simulink model "bpsk_receiver"  (R2020a)
settings: Solver=VariableStepAuto  StartTime=0.0  StopTime=10000/3.2e6  RelTol=1e-3
InitFcn:
  | setup_bpsk_receiver
undefined symbols (not defined in the file): AXI4, designMultirateFIR, fir_bbuf, Lite, tx_data, xlfda_numerator
libraries: xbsIndex_r4 x367, hdlsllib x15, dspmlti4 x8, xrbsSSR_Library x6, dspswit3 x4, dspsigops x2, commrandsrc3 x1, simulink x1
(part 1 of 4)
settings Model: SimulationMode=accelerator  Creator=david  LastModifiedBy=david
settings SFSimCC: CustomCodeUndefinedFunction=UseInterfaceOnly

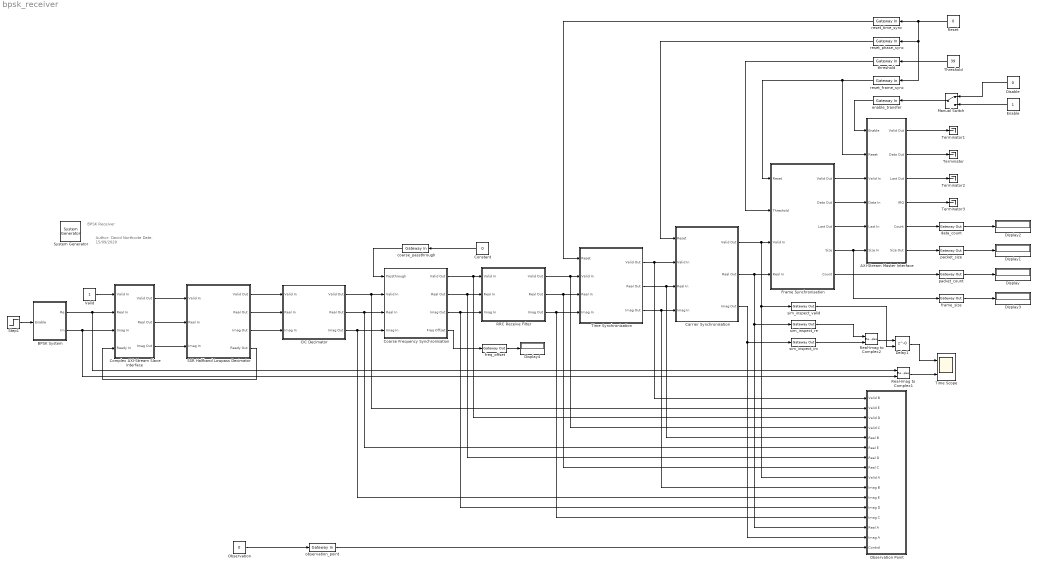
== system bpsk_receiver ==
  note: Author: 	David Northcote
      | Date: 	15/09/2020
  note: BPSK Receiver
  " System Generator" : xbsIndex_r4/ System Generator  Tag=genX  xilinxfamily=zynquplusRFSOC  part=xczu28dr  speed=-2-e  package=ffvg1517  synthesis_tool=Vivado  clock_wrapper=Clock Enables  directory=./netlist  proj_type=Vivado  Synth_file=Vivado Synthesis Defaults  Impl_file=Vivado Implementation Defaults  testbench=off  simulink_period=1/64e6  sysclk_period=(1/64e6)*1e9  dcm_input_clock_period=10  incr_netlist=off  trim_vbits=Everywhere in SubSystem  dbl_ovrd=According to Block Masks  core_generation=According to Block Masks  run_coregen=off  deprecated_control=off  eval_field=0  block_type=sysgen
  AXI-Stream Master Interface : Subsystem
  BPSK System : Subsystem
  CIC Decimator : Subsystem
  Carrier Synchronisation : Subsystem
  Coarse Frequency Synchronisation : Subsystem
  Complex AXI-Stream Slave Interface : Subsystem
  Constant : Constant  Value=0  SampleTime=-1
  Delay1 : Delay  DelayLength=0  ShowEnablePort=on
      settings: InputPortMap=u0,e6
  Disable : Constant  Value=0  OutDataTypeStr=boolean  SampleTime=-1
  Display{,1..4} (5 alike) : Display
  Enable : Constant  OutDataTypeStr=boolean  SampleTime=-1
  Frame Synchronisation : Subsystem
  Manual Switch : ManualSwitch
  Observation : Constant  Value=0  OutDataTypeStr=uint32  SampleTime=-1
  Observation Point : Subsystem
  RRC Receive Filter : Subsystem
  Real-Imag to Complex1 : RealImagToComplex
  Real-Imag to Complex2 : RealImagToComplex
  Reset : Constant  Value=0  OutDataTypeStr=boolean  SampleTime=-1
  SSR Halfband Lowpass Decimator : Subsystem
  Step1 : Step  Time=2/12.5e3  SampleTime=1/12.5e3
  Terminator{,1..3} (4 alike) : Terminator
  Threshold : Constant  Value=39  OutDataTypeStr=uint32  SampleTime=-1
  Time Scope : Scope  NumInputPorts=2
  Time Synchronisation : Subsystem
  Valid : Constant  OutDataTypeStr=boolean  SampleTime=1/64e6
  coarse_passthrough : xbsIndex_r4/Gateway In  gui_display_data_type=Boolean  arith_type=Boolean  n_bits=16  bin_pt=14  preci_type=Single  exp_width=8  frac_width=24  rows=1  columns=1  quantization="Round  (unbiased: +/- Inf)"  overflow=Saturate  period=1/12.8e6  UseAsADC=off  ADCChannel='1'  interface=AXI4-Lite  automatic_assignment=off  address_offset=44  intf_name=''  intf_description=''  default_value=0  timing_constraint=None  locs_specified=off  LOCs={}  io_standard={}  inherit_from_input=off  hdl_port=on  dbl_ovrd=off  block_type=gatewayin
  data_count : xbsIndex_r4/Gateway Out  inherit_from_input=on  hdl_port=on  rows=1  columns=1  UseAsDAC=off  DACChannel='1'  interface=AXI4-Lite  automatic_assignment=off  address_offset=32  intf_name=''  intf_description=''  timing_constraint=None  locs_specified=off  LOCs={}  io_standard={}  block_type=gatewayout
  enable_transfer : xbsIndex_r4/Gateway In  gui_display_data_type=Boolean  arith_type=Boolean  n_bits=16  bin_pt=14  preci_type=Single  exp_width=8  frac_width=24  rows=1  columns=1  quantization="Round  (unbiased: +/- Inf)"  overflow=Saturate  period=1/64e6  UseAsADC=off  ADCChannel='1'  interface=AXI4-Lite  automatic_assignment=off  address_offset=28  intf_name=''  intf_description=''  default_value=0  timing_constraint=None  locs_specified=off  LOCs={}  io_standard={}  inherit_from_input=off  hdl_port=on  dbl_ovrd=off  block_type=gatewayin
  frame_size : xbsIndex_r4/Gateway Out  inherit_from_input=on  hdl_port=on  rows=1  columns=1  UseAsDAC=off  DACChannel='1'  interface=AXI4-Lite  automatic_assignment=off  address_offset=16  intf_name=''  intf_description=''  timing_constraint=None  locs_specified=off  LOCs={}  io_standard={}  block_type=gatewayout
  freq_offset : xbsIndex_r4/Gateway Out  inherit_from_input=on  hdl_port=on  rows=1  columns=1  UseAsDAC=off  DACChannel='1'  interface=AXI4-Lite  automatic_assignment=off  address_offset=40  intf_name=''  intf_description=''  timing_constraint=None  locs_specified=off  LOCs={}  io_standard={}  block_type=gatewayout
  observation_point : xbsIndex_r4/Gateway In  gui_display_data_type=Fixed-point  arith_type=Unsigned  n_bits=32  bin_pt=0  preci_type=Single  exp_width=8  frac_width=24  rows=1  columns=1  quantization="Round  (unbiased: +/- Inf)"  overflow=Saturate  period=1/64e6  UseAsADC=off  ADCChannel='1'  interface=AXI4-Lite  automatic_assignment=off  address_offset=36  intf_name=''  intf_description=''  default_value=0  timing_constraint=None  locs_specified=off  LOCs={}  io_standard={}  inherit_from_input=off  hdl_port=on  dbl_ovrd=off  block_type=gatewayin
  packet_count : xbsIndex_r4/Gateway Out  inherit_from_input=on  hdl_port=on  rows=1  columns=1  UseAsDAC=off  DACChannel='1'  interface=AXI4-Lite  automatic_assignment=off  address_offset=24  intf_name=''  intf_description=''  timing_constraint=None  locs_specified=off  LOCs={}  io_standard={}  block_type=gatewayout
  packet_size : xbsIndex_r4/Gateway Out  inherit_from_input=on  hdl_port=on  rows=1  columns=1  UseAsDAC=off  DACChannel='1'  interface=AXI4-Lite  automatic_assignment=off  address_offset=20  intf_name=''  intf_description=''  timing_constraint=None  locs_specified=off  LOCs={}  io_standard={}  block_type=gatewayout
  reset_frame_sync : xbsIndex_r4/Gateway In  gui_display_data_type=Boolean  arith_type=Boolean  n_bits=16  bin_pt=14  preci_type=Single  exp_width=8  frac_width=24  rows=1  columns=1  quantization="Round  (unbiased: +/- Inf)"  overflow=Saturate  period=1/3.2e6  UseAsADC=off  ADCChannel='1'  interface=AXI4-Lite  automatic_assignment=off  address_offset=8  intf_name=''  intf_description=''  default_value=1  timing_constraint=None  locs_specified=off  LOCs={}  io_standard={}  inherit_from_input=off  hdl_port=on  dbl_ovrd=off  block_type=gatewayin
  reset_phase_sync : xbsIndex_r4/Gateway In  gui_display_data_type=Boolean  arith_type=Boolean  n_bits=16  bin_pt=14  preci_type=Single  exp_width=8  frac_width=24  rows=1  columns=1  quantization="Round  (unbiased: +/- Inf)"  overflow=Saturate  period=1/3.2e6  UseAsADC=off  ADCChannel='1'  interface=AXI4-Lite  automatic_assignment=off  address_offset=4  intf_name=''  intf_description=''  default_value=1  timing_constraint=None  locs_specified=off  LOCs={}  io_standard={}  inherit_from_input=off  hdl_port=on  dbl_ovrd=off  block_type=gatewayin
  reset_time_sync : xbsIndex_r4/Gateway In  gui_display_data_type=Boolean  arith_type=Boolean  n_bits=16  bin_pt=14  preci_type=Single  exp_width=8  frac_width=24  rows=1  columns=1  quantization="Round  (unbiased: +/- Inf)"  overflow=Saturate  period=1/3.2e6  UseAsADC=off  ADCChannel='1'  interface=AXI4-Lite  automatic_assignment=off  address_offset=0  intf_name=''  intf_description=''  default_value=1  timing_constraint=None  locs_specified=off  LOCs={}  io_standard={}  inherit_from_input=off  hdl_port=on  dbl_ovrd=off  block_type=gatewayin
  sim_inspect_im : xbsIndex_r4/Gateway Out  inherit_from_input=on  hdl_port=off  rows=1  columns=1  UseAsDAC=off  DACChannel='1'  interface=None  automatic_assignment=on  address_offset=hex2dec('00')  intf_name=''  intf_description=''  timing_constraint=None  locs_specified=off  LOCs={}  io_standard={}  block_type=gatewayout
  sim_inspect_re : xbsIndex_r4/Gateway Out  inherit_from_input=on  hdl_port=off  rows=1  columns=1  UseAsDAC=off  DACChannel='1'  interface=None  automatic_assignment=on  address_offset=hex2dec('00')  intf_name=''  intf_description=''  timing_constraint=None  locs_specified=off  LOCs={}  io_standard={}  block_type=gatewayout
  sim_inspect_valid : xbsIndex_r4/Gateway Out  inherit_from_input=on  hdl_port=off  rows=1  columns=1  UseAsDAC=off  DACChannel='1'  interface=None  automatic_assignment=on  address_offset=hex2dec('00')  intf_name=''  intf_description=''  timing_constraint=None  locs_specified=off  LOCs={}  io_standard={}  block_type=gatewayout
  threshold : xbsIndex_r4/Gateway In  gui_display_data_type=Fixed-point  arith_type=Unsigned  n_bits=32  bin_pt=0  preci_type=Single  exp_width=8  frac_width=24  rows=1  columns=1  quantization="Round  (unbiased: +/- Inf)"  overflow=Saturate  period=1/3.2e6  UseAsADC=off  ADCChannel='1'  interface=AXI4-Lite  automatic_assignment=off  address_offset=12  intf_name=''  intf_description=''  default_value=39  timing_constraint=None  locs_specified=off  LOCs={}  io_standard={}  inherit_from_input=off  hdl_port=on  dbl_ovrd=off  block_type=gatewayin
  wires:
  reset_time_sync/1 -> Time Synchronisation/1(Reset)
  Reset/1 -> reset_phase_sync/1, reset_frame_sync/1, reset_time_sync/1
  Time Synchronisation/1(Valid Out) -> Observation Point/1(Valid B), Carrier Synchronisation/2(Valid In)
  Time Synchronisation/2(Real Out) -> Carrier Synchronisation/3(Real In), Observation Point/5(Real B)
  Time Synchronisation/3(Imag Out) -> Carrier Synchronisation/4(Imag In), Observation Point/10(Imag B)
  reset_phase_sync/1 -> Carrier Synchronisation/1(Reset)
  Carrier Synchronisation/2(Real Out) -> sim_inspect_re/1, Observation Point/14(Real A), Frame Synchronisation/4(Real In)
  Carrier Synchronisation/1(Valid Out) -> sim_inspect_valid/1, Observation Point/9(Valid A), Frame Synchronisation/3(Valid In)
  threshold/1 -> Frame Synchronisation/2(Threshold)
  reset_frame_sync/1 -> AXI-Stream Master Interface/2(Reset), Frame Synchronisation/1(Reset)
  Threshold/1 -> threshold/1
  Carrier Synchronisation/3(Imag Out) -> sim_inspect_im/1, Observation Point/15(Imag A)
  Frame Synchronisation/5(Count) -> packet_count/1
  Real-Imag to Complex1/1 -> Time Scope/2
  sim_inspect_valid/1 -> Delay1/2
  Real-Imag to Complex2/1 -> Delay1/1
  sim_inspect_re/1 -> Real-Imag to Complex2/1
  sim_inspect_im/1 -> Real-Imag to Complex2/2
  Delay1/1 -> Time Scope/1
  Frame Synchronisation/3(Last Out) -> AXI-Stream Master Interface/5(Last In)
  packet_count/1 -> Display/1
  packet_size/1 -> Display1/1
  AXI-Stream Master Interface/6(Size Out) -> packet_size/1
  Frame Synchronisation/4(Size) -> frame_size/1, AXI-Stream Master Interface/6(Size In)
  enable_transfer/1 -> AXI-Stream Master Interface/1(Enable)
  AXI-Stream Master Interface/5(Count) -> data_count/1
  data_count/1 -> Display2/1
  AXI-Stream Master Interface/2(Data Out) -> Terminator/1
  AXI-Stream Master Interface/1(Valid Out) -> Terminator1/1
  AXI-Stream Master Interface/3(Last Out) -> Terminator2/1
  AXI-Stream Master Interface/4(IRQ) -> Terminator3/1
  Frame Synchronisation/1(Valid Out) -> AXI-Stream Master Interface/3(Valid In)
  Frame Synchronisation/2(Data Out) -> AXI-Stream Master Interface/4(Data In)
  Manual Switch/1 -> enable_transfer/1
  Disable/1 -> Manual Switch/1
  Enable/1 -> Manual Switch/2
  Complex AXI-Stream Slave Interface/3(Imag Out) -> SSR Halfband Lowpass Decimator/3(Imag In)
  Complex AXI-Stream Slave Interface/2(Real Out) -> SSR Halfband Lowpass Decimator/2(Real In)
  Complex AXI-Stream Slave Interface/1(Valid Out) -> SSR Halfband Lowpass Decimator/1(Valid In)
  SSR Halfband Lowpass Decimator/4(Ready Out) -> Complex AXI-Stream Slave Interface/4(Ready In)
  Valid/1 -> Complex AXI-Stream Slave Interface/1(Valid In)
  Step1/1 -> BPSK System/1(Enable)
  BPSK System/2(Im) -> Complex AXI-Stream Slave Interface/3(Imag In), Real-Imag to Complex1/2
  BPSK System/1(Re) -> Complex AXI-Stream Slave Interface/2(Real In), Real-Imag to Complex1/1
  RRC Receive Filter/1(Valid Out) -> Time Synchronisation/2(Valid In), Observation Point/4(Valid C)
  RRC Receive Filter/2(Real Out) -> Time Synchronisation/3(Real In), Observation Point/8(Real C)
  RRC Receive Filter/3(Imag Out) -> Time Synchronisation/4(Imag In), Observation Point/13(Imag C)
  SSR Halfband Lowpass Decimator/2(Real Out) -> CIC Decimator/2(Real In)
  SSR Halfband Lowpass Decimator/3(Imag Out) -> CIC Decimator/3(Imag In)
  Observation/1 -> observation_point/1
  observation_point/1 -> Observation Point/16(Control)
  frame_size/1 -> Display3/1
  CIC Decimator/1(Valid Out) -> Coarse Frequency Synchronisation/2(Valid In), Observation Point/2(Valid E)
  CIC Decimator/2(Real Out) -> Coarse Frequency Synchronisation/3(Real In), Observation Point/6(Real E)
  CIC Decimator/3(Imag Out) -> Coarse Frequency Synchronisation/4(Imag In), Observation Point/11(Imag E)
  Coarse Frequency Synchronisation/1(Valid Out) -> Observation Point/3(Valid D), RRC Receive Filter/1(Valid In)
  Coarse Frequency Synchronisation/2(Real Out) -> Observation Point/7(Real D), RRC Receive Filter/2(Real In)
  Coarse Frequency Synchronisation/3(Imag Out) -> Observation Point/12(Imag D), RRC Receive Filter/3(Imag In)
  freq_offset/1 -> Display4/1
  Coarse Frequency Synchronisation/4(Freq Offset) -> freq_offset/1
  Constant/1 -> coarse_passthrough/1
  coarse_passthrough/1 -> Coarse Frequency Synchronisation/1(Passthrough)
  SSR Halfband Lowpass Decimator/1(Valid Out) -> CIC Decimator/1(Valid In)

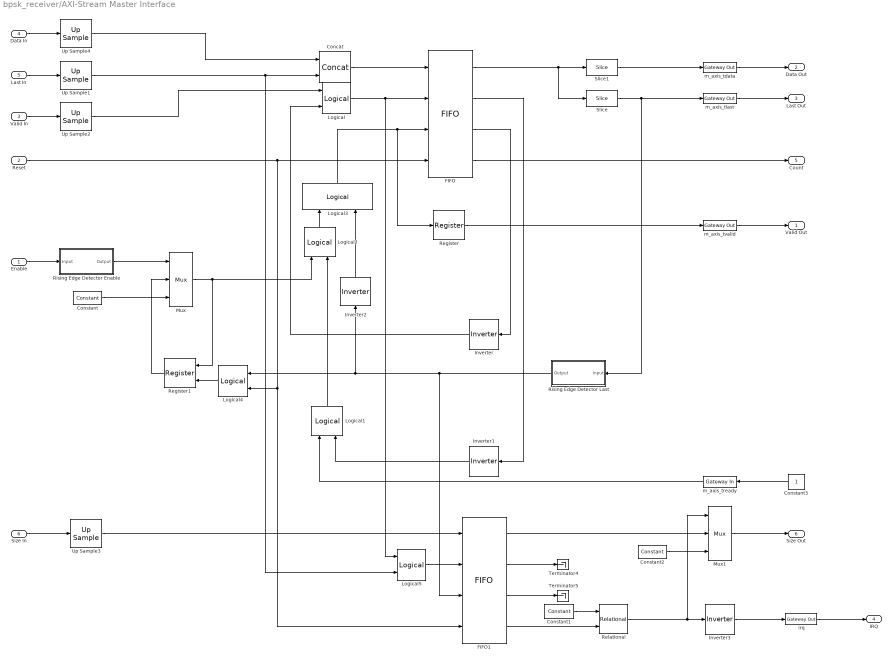
== system bpsk_receiver/AXI-Stream Master Interface ==
  Enable : Inport
  Reset : Inport  Port=2
  Valid In : Inport  Port=3
  Data In : Inport  Port=4
  Last In : Inport  Port=5
  Size In : Inport  Port=6
  Concat : xbsIndex_r4/Concat  num_inputs=2  dbl_ovrd=off  block_type=concat
  Constant : xbsIndex_r4/Constant  const=1.0  gui_display_data_type=Boolean  arith_type=Boolean  n_bits=16  bin_pt=14  preci_type=Single  exp_width=8  frac_width=24  explicit_period=off  period=1  equ=P=C  opselect=C  inp2=PCIN>>17  opr=+  inp1=P  carry=CIN  dbl_ovrd=off  block_type=constant
  Constant1 : xbsIndex_r4/Constant  const=0  gui_display_data_type=Fixed-point  arith_type=Unsigned  n_bits=1  bin_pt=0  preci_type=Single  exp_width=8  frac_width=24  explicit_period=off  period=1  equ=P=C  opselect=C  inp2=PCIN>>17  opr=+  inp1=P  carry=CIN  dbl_ovrd=off  block_type=constant
  Constant2 : xbsIndex_r4/Constant  const=0  gui_display_data_type=Fixed-point  arith_type=Unsigned  n_bits=8  bin_pt=0  preci_type=Single  exp_width=8  frac_width=24  explicit_period=off  period=1  equ=P=C  opselect=C  inp2=PCIN>>17  opr=+  inp1=P  carry=CIN  dbl_ovrd=off  block_type=constant
  Constant3 : Constant  SampleTime=1/64e6
  FIFO : xbsIndex_r4/FIFO  mem_type=Block RAM  performance_options=Standard_FIFO  embedded_registers=off  depth=4K  percent_nbits=1  rst=on  rst_latency=2  en=off  use_dcount=on  use_percent_full_port=off  use_almost_empty=off  almost_empty_thresh=2  use_almost_full=off  use_rd_rst_busy=off  use_wr_rst_busy=off  almost_full_thresh=14  explicit_period=off  dbl_ovrd=off  simulation_type=fast_sim  block_type=fifo
  FIFO1 : xbsIndex_r4/FIFO  mem_type=Block RAM  performance_options=First_Word_Fall_Through  embedded_registers=off  depth=4K  percent_nbits=1  rst=on  rst_latency=2  en=off  use_dcount=on  use_percent_full_port=off  use_almost_empty=off  almost_empty_thresh=2  use_almost_full=off  use_rd_rst_busy=off  use_wr_rst_busy=off  almost_full_thresh=14  explicit_period=off  dbl_ovrd=off  simulation_type=fast_sim  block_type=fifo
  Inverter{,1..3} (4 alike) : xbsIndex_r4/Inverter  en=off  latency=0  dbl_ovrd=off  block_type=inv
  Logical{,1..3,5} (5 alike) : xbsIndex_r4/Logical  logical_function=AND  inputs=2  en=off  latency=0  precision=Full  arith_type=Unsigned  n_bits=16  bin_pt=0  align_bp=on  dbl_ovrd=off  block_type=logical
  Logical4 : xbsIndex_r4/Logical  logical_function=OR  inputs=2  en=off  latency=0  precision=Full  arith_type=Unsigned  n_bits=16  bin_pt=0  align_bp=on  dbl_ovrd=off  block_type=logical
  Mux : xbsIndex_r4/Mux  inputs=2  en=off  latency=0  precision=Full  arith_type=Unsigned  n_bits=16  bin_pt=14  quantization=Truncate  overflow=Wrap  dbl_ovrd=off  block_type=mux
  Mux1 : xbsIndex_r4/Mux  inputs=2  en=off  latency=0  precision=Full  arith_type=Unsigned  n_bits=16  bin_pt=14  quantization=Truncate  overflow=Wrap  dbl_ovrd=off  block_type=mux
  Register : xbsIndex_r4/Register  init=0  rst=off  en=off  dbl_ovrd=off  block_type=register
  Register1 : xbsIndex_r4/Register  init=0  rst=on  en=off  dbl_ovrd=off  block_type=register
  Relational : xbsIndex_r4/Relational  mode=a=b  op_type=Bool  en=off  latency=0  dbl_ovrd=off  block_type=relational
  Rising Edge Detector Enable : Subsystem
  Rising Edge Detector Last : Subsystem
  Slice : xbsIndex_r4/Slice  nbits=1  boolean_output=on  mode=Two Bit Locations  bit1=0  base1=LSB of Input  bit0=0  base0=LSB of Input  dbl_ovrd=off  block_type=slice
  Slice1 : xbsIndex_r4/Slice  nbits=1  boolean_output=off  mode=Two Bit Locations  bit1=8  base1=LSB of Input  bit0=1  base0=LSB of Input  dbl_ovrd=off  block_type=slice
  Terminator4 : Terminator
  Terminator5 : Terminator
  Up Sample{1..4} (4 alike) : xbsIndex_r4/Up Sample  sample_ratio=64e6/3.2e6  copy_samples=off  en=off  latency=1  dbl_ovrd=off  block_type=usamp
  irq : xbsIndex_r4/Gateway Out  inherit_from_input=on  hdl_port=on  rows=1  columns=1  UseAsDAC=off  DACChannel='1'  interface=Interrupt  automatic_assignment=off  address_offset=36  intf_name=''  intf_description=''  timing_constraint=None  locs_specified=off  LOCs={}  io_standard={}  block_type=gatewayout
  m_axis_tdata : xbsIndex_r4/Gateway Out  inherit_from_input=on  hdl_port=on  rows=1  columns=1  UseAsDAC=off  DACChannel='1'  interface=None  automatic_assignment=on  address_offset=hex2dec('00')  intf_name=''  intf_description=''  timing_constraint=None  locs_specified=off  LOCs={}  io_standard={}  block_type=gatewayout
  m_axis_tlast : xbsIndex_r4/Gateway Out  inherit_from_input=on  hdl_port=on  rows=1  columns=1  UseAsDAC=off  DACChannel='1'  interface=None  automatic_assignment=on  address_offset=hex2dec('00')  intf_name=''  intf_description=''  timing_constraint=None  locs_specified=off  LOCs={}  io_standard={}  block_type=gatewayout
  m_axis_tready : xbsIndex_r4/Gateway In  gui_display_data_type=Boolean  arith_type=Boolean  n_bits=16  bin_pt=14  preci_type=Single  exp_width=8  frac_width=24  rows=1  columns=1  quantization="Round  (unbiased: +/- Inf)"  overflow=Saturate  period=1/64e6  UseAsADC=off  ADCChannel='1'  interface=None  automatic_assignment=on  address_offset=hex2dec('00')  intf_name=''  intf_description=''  default_value=0  timing_constraint=None  locs_specified=off  LOCs={}  io_standard={}  inherit_from_input=off  hdl_port=on  dbl_ovrd=off  block_type=gatewayin
  m_axis_tvalid : xbsIndex_r4/Gateway Out  inherit_from_input=on  hdl_port=on  rows=1  columns=1  UseAsDAC=off  DACChannel='1'  interface=None  automatic_assignment=on  address_offset=hex2dec('00')  intf_name=''  intf_description=''  timing_constraint=None  locs_specified=off  LOCs={}  io_standard={}  block_type=gatewayout
  Valid Out : Outport  VectorParamsAs1DForOutWhenUnconnected=off
  Data Out : Outport  Port=2  VectorParamsAs1DForOutWhenUnconnected=off
  Last Out : Outport  Port=3  VectorParamsAs1DForOutWhenUnconnected=off
  IRQ : Outport  Port=4  VectorParamsAs1DForOutWhenUnconnected=off
  Count : Outport  Port=5  VectorParamsAs1DForOutWhenUnconnected=off
  Size Out : Outport  Port=6  VectorParamsAs1DForOutWhenUnconnected=off
  wires:
  irq/1 -> IRQ/1
  Constant3/1 -> m_axis_tready/1
  Up Sample3/1 -> FIFO1/1
  Up Sample2/1 -> Logical/1
  Up Sample1/1 -> Logical5/2, Concat/2
  Up Sample4/1 -> Concat/1
  m_axis_tvalid/1 -> Valid Out/1
  m_axis_tlast/1 -> Last Out/1
  m_axis_tdata/1 -> Data Out/1
  FIFO/1 -> Slice1/1, Slice/1
  Logical/1 -> Logical5/1, FIFO/2
  Valid In/1 -> Up Sample2/1
  FIFO/3 -> Inverter/1
  Inverter/1 -> Logical/2
  FIFO/2 -> Inverter1/1
  Inverter1/1 -> Logical1/2
  m_axis_tready/1 -> Logical1/1
  Concat/1 -> FIFO/1
  Last In/1 -> Up Sample1/1
  Data In/1 -> Up Sample4/1
  FIFO/4 -> Count/1
  Slice1/1 -> m_axis_tdata/1
  Register/1 -> m_axis_tvalid/1
  Logical1/1 -> Logical2/2
  Mux/1 -> Register1/1, Logical2/1
  Rising Edge Detector Enable/1(Output) -> Mux/1
  Register1/1 -> Mux/2
  Constant/1 -> Mux/3
  Enable/1 -> Rising Edge Detector Enable/1(Input)
  Slice/1 -> Rising Edge Detector Last/1(Input), m_axis_tlast/1
  Rising Edge Detector Last/1(Output) -> FIFO1/3, Inverter2/1, Logical4/1
  Logical3/1 -> FIFO/3, Register/1
  Logical2/1 -> Logical3/1
  Inverter2/1 -> Logical3/2
  Logical4/1 -> Register1/2
  Size In/1 -> Up Sample3/1
  FIFO1/2 -> Terminator4/1
  FIFO1/3 -> Terminator5/1
  FIFO1/4 -> Relational/2
  Logical5/1 -> FIFO1/2
  Constant1/1 -> Relational/1
  FIFO1/1 -> Mux1/2
  Mux1/1 -> Size Out/1
  Relational/1 -> Inverter3/1, Mux1/1
  Constant2/1 -> Mux1/3
  Inverter3/1 -> irq/1
  Reset/1 -> FIFO/4, Logical4/2, FIFO1/4

== system bpsk_receiver/BPSK System ==
  Enable : Inport
  BPSK TX Generation : Subsystem
  Complex to Real-Imag : ComplexToRealImag
  RF Balun Gain RX : Gain  Gain=1/2
  RF Balun Gain TX : Gain  Gain=1/2
  RF-ADC : Subsystem  mask{fs_ghz=1.024, decim=8x, ssr=2, mode=Fine, fc=0.064100, fph=0, fcoarse=fs/4}
      mask prompts: fs_ghz "Sample Rate (GHz):"; decim "Interpolation Mode:"; ssr "Samples per AXI4-Stream Cycle:"; mode "Mixer Type:"; fc "NCO Frequency (GHz):"; fph "NCO Phase (Rads):"; fcoarse "Frequency:"
      mask init:
      | % Obtain the sample rate in Hz
      | fs = str2double(get_param(gcb, 'fs_ghz'))*1e9;
      | 
      | % Set the mode of the RF-DAC interpolation filter
      | switch get_param(gcb, 'decim')
      |     case '1x'
      |         D = 1;
      |     case '2x'
      |         D = 2;
      |     case '4x'
      |         D = 4;
      |     case '8x'
      |         D = 8;
      |     otherwise
      |         D = 1;
      | end
      | 
      | % Get the AXI-Stream clock for display to user
      | axi_clk = (fs/(str2double(get_param(gcb, 'ssr'))*D))*1e-6;
      | 
      | % Get the block mask object to manipulate settings
      | mo = get_param(gcb, 'MaskObject');
      | 
      | % Update text to display the required AXI-Stream clock
      | tc = mo.getDialogControl('axi_text');
      | tc.Prompt = ['      Required AXI-Stream Clock: ', num2str(axi_clk), ' MHz'];
      | 
      | % Set the RF-DAC Mixer mode
      | switch get_param(gcb, 'mode')
      |     case 'Bypass'
      |         m = 0;
      |     case 'Coarse'
      |         m = 1;
      |     case 'Fine'
      |         m = 2;
      |     otherwise
      |         m = 0;
      | end
      | 
      | % Set the RF-DAC Coarse Mixer mode
      | switch get_param(gcb, 'fcoarse')
      |     case 'fs/2'
      |         mc = 0;
      |     case 'fs/4'
      |         mc = 1;
      |     case '-fs/4'
      |         mc = 2;
      |     otherwise
      |         mc = 0;
      | end
      | 
      | % Set other blocks
      | set_param([gcb, '/Decimation Filter'], 'decim', get_param(gcb, 'decim'));
      mask Callback fs_ghz:
      | % Obtain the sample rate in Hz
      | fs = str2double(get_param(gcb, 'fs_ghz'))*1e9;
      | 
      | % Set the mode of the RF-DAC interpolation filter
      | switch get_param(gcb, 'decim')
      |     case '1x'
      |         D = 1;
      |     case '2x'
      |         D = 2;
      |     case '4x'
      |         D = 4;
      |     case '8x'
      |         D = 8;
      |     otherwise
      |         D = 1;
      | end
      | 
      | % Get the AXI-Stream clock for display to user
      | axi_clk = (fs/(str2double(get_param(gcb, 'ssr'))*D))*1e-6;
      | 
      | % Get the block mask object to manipulate settings
      | mo = get_param(gcb, 'MaskObject');
      | 
      | % Update text to display the required AXI-Stream clock
      | tc = mo.getDialogControl('axi_text');
      | tc.Prompt = ['      Required AXI-Stream Clock: ', num2str(axi_clk), ' MHz'];
      mask TypeOptions decim: 1x | 2x | 4x | 8x
      mask Callback decim:
      | % Obtain the sample rate in Hz
      | fs = str2double(get_param(gcb, 'fs_ghz'))*1e9;
      | 
      | % Set the mode of the RF-DAC interpolation filter
      | switch get_param(gcb, 'decim')
      |     case '1x'
      |         D = 1;
      |     case '2x'
      |         D = 2;
      |     case '4x'
      |         D = 4;
      |     case '8x'
      |         D = 8;
      |     otherwise
      |         D = 1;
      | end
      | 
      | % Get the AXI-Stream clock for display to user
      | axi_clk = (fs/(str2double(get_param(gcb, 'ssr'))*D))*1e-6;
      | 
      | % Get the block mask object to manipulate settings
      | mo = get_param(gcb, 'MaskObject');
      | 
      | % Update text to display the required AXI-Stream clock
      | tc = mo.getDialogControl('axi_text');
      | tc.Prompt = ['      Required AXI-Stream Clock: ', num2str(axi_clk), ' MHz'];
      mask TypeOptions ssr: 1 | 2 | 3 | 4 | 5 | 6 | 7 | 8 | 9 | 10 | 11 | 12 | 13 | 14 | 15 | 16
      mask Callback ssr:
      | % Obtain the sample rate in Hz
      | fs = str2double(get_param(gcb, 'fs_ghz'))*1e9;
      | 
      | % Set the mode of the RF-DAC interpolation filter
      | switch get_param(gcb, 'decim')
      |     case '1x'
      |         D = 1;
      |     case '2x'
      |         D = 2;
      |     case '4x'
      |         D = 4;
      |     case '8x'
      |         D = 8;
      |     otherwise
      |         D = 1;
      | end
      | 
      | % Get the AXI-Stream clock for display to user
      | axi_clk = (fs/(str2double(get_param(gcb, 'ssr'))*D))*1e-6;
      | 
      | % Get the block mask object to manipulate settings
      | mo = get_param(gcb, 'MaskObject');
      | 
      | % Update text to display the required AXI-Stream clock
      | tc = mo.getDialogControl('axi_text');
      | tc.Prompt = ['      Required AXI-Stream Clock: ', num2str(axi_clk), ' MHz'];
      mask TypeOptions mode: Coarse | Fine
      mask Callback mode:
      | % Get the block mask object to manipulate settings
      | mo = get_param(gcb, 'MaskObject');
      | 
      | % Hide group depending on Mixer mode choice
      | switch get_param(gcb, 'mode')
      |     case 'Bypass'
      |         mo.getDialogControl('coarse_group').Visible='off';
      |         mo.getDialogControl('mixer_group').Visible='off';
      |     case 'Coarse'
      |         mo.getDialogControl('coarse_group').Visible='on';
      |         mo.getDialogControl('mixer_group').Visible='off';
      |     case 'Fine'
      |         mo.getDialogControl('coarse_group').Visible='off';
      |         mo.getDialogControl('mixer_group').Visible='on';
      |     otherwise
      |         mo.getDialogControl('coarse_group').Visible='off';
      |         mo.getDialogControl('mixer_group').Visible='off';
      | end
      mask TypeOptions fcoarse: fs/2 | fs/4 | -fs/4
      mask DialogControl DescGroupVar Prompt: RF-DAC
      mask DialogControl DescTextVar Prompt: This block simulates one RF-ADC channel.
      mask DialogControl main_group Prompt: Data Settings
      mask DialogControl axi_text Prompt: Required AXI-Stream Clock: 64 MHz
      mask DialogControl Container5 Prompt: Mixer Settings
  RF-DAC : Subsystem  mask{fs_ghz=1.024, interp=8x, ssr=1, mode=Fine, fc=0.064, fph=0, fcoarse=fs/4}
      mask prompts: fs_ghz "Sample Rate (GHz):"; interp "Interpolation Mode:"; ssr "Samples per AXI4-Stream Cycle:"; mode "Mixer Type:"; fc "NCO Frequency (GHz):"; fph "NCO Phase (Rads):"; fcoarse "Frequency:"
      mask init:
      | % Obtain the sample rate in Hz
      | fs = str2double(get_param(gcb, 'fs_ghz'))*1e9;
      | 
      | % Set the mode of the RF-DAC interpolation filter
      | switch get_param(gcb, 'interp')
      |     case '1x'
      |         L = 1;
      |     case '2x'
      |         L = 2;
      |     case '4x'
      |         L = 4;
      |     case '8x'
      |         L = 8;
      |     otherwise
      |         L = 1;
      | end
      | 
      | % Get the AXI-Stream clock for display to user
      | axi_clk = (fs/(str2double(get_param(gcb, 'ssr'))*L))*1e-6;
      | 
      | % Get the block mask object to manipulate settings
      | mo = get_param(gcb, 'MaskObject');
      | 
      | % Update text to display the required AXI-Stream clock
      | tc = mo.getDialogControl('axi_text');
      | tc.Prompt = ['      Required AXI-Stream Clock: ', num2str(axi_clk), ' MHz'];
      | 
      | % Set the RF-DAC Mixer mode
      | switch get_param(gcb, 'mode')
      |     case 'Bypass'
      |         m = 0;
      |     case 'Coarse'
      |         m = 1;
      |     case 'Fine'
      |         m = 2;
      |     otherwise
      |         m = 0;
      | end
      | 
      | % Set the RF-DAC Coarse Mixer mode
      | switch get_param(gcb, 'fcoarse')
      |     case 'fs/2'
      |         mc = 0;
      |     case 'fs/4'
      |         mc = 1;
      |     case '-fs/4'
      |         mc = 2;
      |     otherwise
      |         mc = 0;
      | end
      | 
      | % Set other blocks
      | set_param([gcb, '/Interpolation Filter'], 'interp', get_param(gcb, 'interp'));
      mask Callback fs_ghz:
      | % Obtain the sample rate in Hz
      | fs = str2double(get_param(gcb, 'fs_ghz'))*1e9;
      | 
      | % Set the mode of the RF-DAC interpolation filter
      | switch get_param(gcb, 'interp')
      |     case '1x'
      |         L = 1;
      |     case '2x'
      |         L = 2;
      |     case '4x'
      |         L = 4;
      |     case '8x'
      |         L = 8;
      |     otherwise
      |         L = 1;
      | end
      | 
      | % Get the AXI-Stream clock for display to user
      | axi_clk = (fs/(str2double(get_param(gcb, 'ssr'))*L))*1e-6;
      | 
      | % Get the block mask object to manipulate settings
      | mo = get_param(gcb, 'MaskObject');
      | 
      | % Update text to display the required AXI-Stream clock
      | tc = mo.getDialogControl('axi_text');
      | tc.Prompt = ['      Required AXI-Stream Clock: ', num2str(axi_clk), ' MHz'];
      mask TypeOptions interp: 1x | 2x | 4x | 8x
      mask Callback interp:
      | % Obtain the sample rate in Hz
      | fs = str2double(get_param(gcb, 'fs_ghz'))*1e9;
      | 
      | % Set the mode of the RF-DAC interpolation filter
      | switch get_param(gcb, 'interp')
      |     case '1x'
      |         L = 1;
      |     case '2x'
      |         L = 2;
      |     case '4x'
      |         L = 4;
      |     case '8x'
      |         L = 8;
      |     otherwise
      |         L = 1;
      | end
      | 
      | % Get the AXI-Stream clock for display to user
      | axi_clk = (fs/(str2double(get_param(gcb, 'ssr'))*L))*1e-6;
      | 
      | % Get the block mask object to manipulate settings
      | mo = get_param(gcb, 'MaskObject');
      | 
      | % Update text to display the required AXI-Stream clock
      | tc = mo.getDialogControl('axi_text');
      | tc.Prompt = ['      Required AXI-Stream Clock: ', num2str(axi_clk), ' MHz'];
      mask TypeOptions ssr: 1 | 2 | 3 | 4 | 5 | 6 | 7 | 8 | 9 | 10 | 11 | 12 | 13 | 14 | 15 | 16
      mask Callback ssr:
      | % Obtain the sample rate in Hz
      | fs = str2double(get_param(gcb, 'fs_ghz'))*1e9;
      | 
      | % Set the mode of the RF-DAC interpolation filter
      | switch get_param(gcb, 'interp')
      |     case '1x'
      |         L = 1;
      |     case '2x'
      |         L = 2;
      |     case '4x'
      |         L = 4;
      |     case '8x'
      |         L = 8;
      |     otherwise
      |         L = 1;
      | end
      | 
      | % Get the AXI-Stream clock for display to user
      | axi_clk = (fs/(str2double(get_param(gcb, 'ssr'))*L))*1e-6;
      | 
      | % Get the block mask object to manipulate settings
      | mo = get_param(gcb, 'MaskObject');
      | 
      | % Update text to display the required AXI-Stream clock
      | tc = mo.getDialogControl('axi_text');
      | tc.Prompt = ['      Required AXI-Stream Clock: ', num2str(axi_clk), ' MHz'];
      mask TypeOptions mode: Coarse | Fine
      mask Callback mode:
      | % Get the block mask object to manipulate settings
      | mo = get_param(gcb, 'MaskObject');
      | 
      | % Hide group depending on Mixer mode choice
      | switch get_param(gcb, 'mode')
      |     case 'Bypass'
      |         mo.getDialogControl('coarse_group').Visible='off';
      |         mo.getDialogControl('mixer_group').Visible='off';
      |     case 'Coarse'
      |         mo.getDialogControl('coarse_group').Visible='on';
      |         mo.getDialogControl('mixer_group').Visible='off';
      |     case 'Fine'
      |         mo.getDialogControl('coarse_group').Visible='off';
      |         mo.getDialogControl('mixer_group').Visible='on';
      |     otherwise
      |         mo.getDialogControl('coarse_group').Visible='off';
      |         mo.getDialogControl('mixer_group').Visible='off';
      | end
      mask TypeOptions fcoarse: fs/2 | fs/4 | -fs/4
      mask DialogControl DescGroupVar Prompt: RF-DAC
      mask DialogControl DescTextVar Prompt: This block simulates one RF-DAC channel.
      mask DialogControl main_group Prompt: Data Settings
      mask DialogControl axi_text Prompt: Required AXI-Stream Clock: 128 MHz
      mask DialogControl Container5 Prompt: Mixer Settings
  Re : Outport  VectorParamsAs1DForOutWhenUnconnected=off
  Im : Outport  Port=2  VectorParamsAs1DForOutWhenUnconnected=off
  wires:
  BPSK TX Generation/1(BPSK) -> RF-DAC/1(Data In)
  Enable/1 -> BPSK TX Generation/1(Enable)
  Complex to Real-Imag/1 -> Re/1
  Complex to Real-Imag/2 -> Im/1
  RF-ADC/1(Data Out) -> Complex to Real-Imag/1
  RF-DAC/1(Data Out) -> RF Balun Gain TX/1
  RF Balun Gain TX/1 -> RF Balun Gain RX/1
  RF Balun Gain RX/1 -> RF-ADC/1(Data In)

== system bpsk_receiver/CIC Decimator ==
  Valid In : Inport
  Real In : Inport  Port=2
  Imag In : Inport  Port=3
  CIC Decimator Imag : xbsIndex_r4/CIC Compiler 4.0   filter_type=Decimation  number_of_stages=3  differential_delay=1  number_of_channels=1  sample_rate_changes=Fixed  fixed_or_initial_rate=(64e6)/(12.8e6)  minimum_rate=5  maximum_rate=5  ratespecification=Maximum_Possible  sampleperiod=1  hardwareoversamplingrate=1  quantization=Full_Precision  output_data_width=25  use_xtreme_dsp_slice=on  use_streaming_interface=on  has_aclken=off  has_aresetn=off  has_dout_tready=off  trim_axipin_name=on  gui_behaviour=Sysgen_GUI  input_data_width=18  ip_name=CIC Compiler  ip_version=4.0  dsptool_ready=true  wrapper_available=true  port_translation_map={ 'aclken' => 'en', 'aresetn' => 'rst' }  ipcore_xco_need_fpga_part=true  ipcore_verbose=false  block_type=cic_compiler_v4_0
  CIC Decimator Real : xbsIndex_r4/CIC Compiler 4.0   filter_type=Decimation  number_of_stages=3  differential_delay=1  number_of_channels=1  sample_rate_changes=Fixed  fixed_or_initial_rate=(64e6)/(12.8e6)  minimum_rate=5  maximum_rate=5  ratespecification=Maximum_Possible  sampleperiod=1  hardwareoversamplingrate=1  quantization=Full_Precision  output_data_width=25  use_xtreme_dsp_slice=on  use_streaming_interface=on  has_aclken=off  has_aresetn=off  has_dout_tready=off  trim_axipin_name=on  gui_behaviour=Sysgen_GUI  input_data_width=18  ip_name=CIC Compiler  ip_version=4.0  dsptool_ready=true  wrapper_available=true  port_translation_map={ 'aclken' => 'en', 'aresetn' => 'rst' }  ipcore_xco_need_fpga_part=true  ipcore_verbose=false  block_type=cic_compiler_v4_0
  CMult1 : xbsIndex_r4/CMult  const=(2^(floor(log2(((64e6)/(12.8e6))^3))))/(((64e6)/(12.8e6))^3)  gui_display_data_type=Fixed-point  const_n_bits=16  const_bin_pt=14  float_type=Single  exp_bits=8  fraction_bits=24  en=off  latency=1  precision=User Defined  arith_type="Signed  (2's comp)"  n_bits=16  bin_pt=14  quantization=Truncate  overflow=Wrap  use_behavioral_HDL=off  mem_type=Distributed RAM  pipeline=off  dbl_ovrd=off  block_type=cmult
  CMult2 : xbsIndex_r4/CMult  const=(2^(floor(log2(((64e6)/(12.8e6))^3))))/(((64e6)/(12.8e6))^3)  gui_display_data_type=Fixed-point  const_n_bits=16  const_bin_pt=14  float_type=Single  exp_bits=8  fraction_bits=24  en=off  latency=1  precision=User Defined  arith_type="Signed  (2's comp)"  n_bits=16  bin_pt=14  quantization=Truncate  overflow=Wrap  use_behavioral_HDL=off  mem_type=Distributed RAM  pipeline=off  dbl_ovrd=off  block_type=cmult
  Shift1 : xbsIndex_r4/Shift  shift_dir=Right  shift_bits=floor(log2(((64e6)/(12.8e6))^3))  en=off  latency=0  precision=User Defined  arith_type="Signed  (2's comp)"  n_bits=16+ceil(log2(((64e6)/(12.8e6))^3))  bin_pt=16+ceil(log2(((64e6)/(12.8e6))^3))-2  quantization=Truncate  overflow=Wrap  dbl_ovrd=off  block_type=shift
  Shift2 : xbsIndex_r4/Shift  shift_dir=Right  shift_bits=floor(log2(((64e6)/(12.8e6))^3))  en=off  latency=0  precision=User Defined  arith_type="Signed  (2's comp)"  n_bits=16+ceil(log2(((64e6)/(12.8e6))^3))  bin_pt=16+ceil(log2(((64e6)/(12.8e6))^3))-2  quantization=Truncate  overflow=Wrap  dbl_ovrd=off  block_type=shift
  Terminator{1..4} (4 alike) : Terminator
  Valid Out : Outport  VectorParamsAs1DForOutWhenUnconnected=off
  Real Out : Outport  Port=2  VectorParamsAs1DForOutWhenUnconnected=off
  Imag Out : Outport  Port=3  VectorParamsAs1DForOutWhenUnconnected=off
  wires:
  CIC Decimator Real/2 -> Valid Out/1
  Valid In/1 -> Terminator4/1
  Shift2/1 -> CMult2/1
  CIC Decimator Real/3 -> Shift2/1
  CIC Decimator Real/1 -> Terminator2/1
  Real In/1 -> CIC Decimator Real/1
  CMult2/1 -> Real Out/1
  CMult1/1 -> Imag Out/1
  Imag In/1 -> CIC Decimator Imag/1
  CIC Decimator Imag/2 -> Terminator1/1
  CIC Decimator Imag/1 -> Terminator3/1
  CIC Decimator Imag/3 -> Shift1/1
  Shift1/1 -> CMult1/1

== system bpsk_receiver/Carrier Synchronisation ==
  Reset : Inport
  Valid In : Inport  Port=2
  Real In : Inport  Port=3
  Imag In : Inport  Port=4
  Convert : xbsIndex_r4/Convert  gui_display_data_type=Fixed-point  arith_type="Signed  (2's comp)"  n_bits=16  bin_pt=14  float_type=Single  exp_bits=8  fraction_bits=24  quantization=Truncate  overflow=Wrap  en=off  latency=0  pipeline=off  dbl_ovrd=off  block_type=convert
  Convert1 : xbsIndex_r4/Convert  gui_display_data_type=Fixed-point  arith_type="Signed  (2's comp)"  n_bits=16  bin_pt=14  float_type=Single  exp_bits=8  fraction_bits=24  quantization=Truncate  overflow=Wrap  en=off  latency=0  pipeline=off  dbl_ovrd=off  block_type=convert
  De-Rotate Constellation : Subsystem
  Generate Angle Error : Subsystem
  Generate NCO : Subsystem
  Valid Out : Outport  VectorParamsAs1DForOutWhenUnconnected=off
  Real Out : Outport  Port=2  VectorParamsAs1DForOutWhenUnconnected=off
  Imag Out : Outport  Port=3  VectorParamsAs1DForOutWhenUnconnected=off
  wires:
  Reset/1 -> Generate NCO/3(Reset)
  De-Rotate Constellation/1(Imag Out) -> Convert/1
  De-Rotate Constellation/2(Real Out) -> Convert1/1
  De-Rotate Constellation/3(Valid Out) -> Valid Out/1, Generate Angle Error/3(Valid In)
  Generate NCO/3(Valid Out) -> De-Rotate Constellation/6(Valid Error)
  Generate NCO/2(Real Out) -> De-Rotate Constellation/5(Real Error)
  Generate NCO/1(Imag Out) -> De-Rotate Constellation/4(Imag Error)
  Generate Angle Error/1(Angle) -> Generate NCO/1(Angle)
  Generate Angle Error/2(Valid Out) -> Generate NCO/2(Valid In)
  Valid In/1 -> De-Rotate Constellation/3(Valid In)
  Real In/1 -> De-Rotate Constellation/2(Real In)
  Imag In/1 -> De-Rotate Constellation/1(Imag In)
  Convert/1 -> Imag Out/1, Generate Angle Error/1(Imag In)
  Convert1/1 -> Real Out/1, Generate Angle Error/2(Real In)

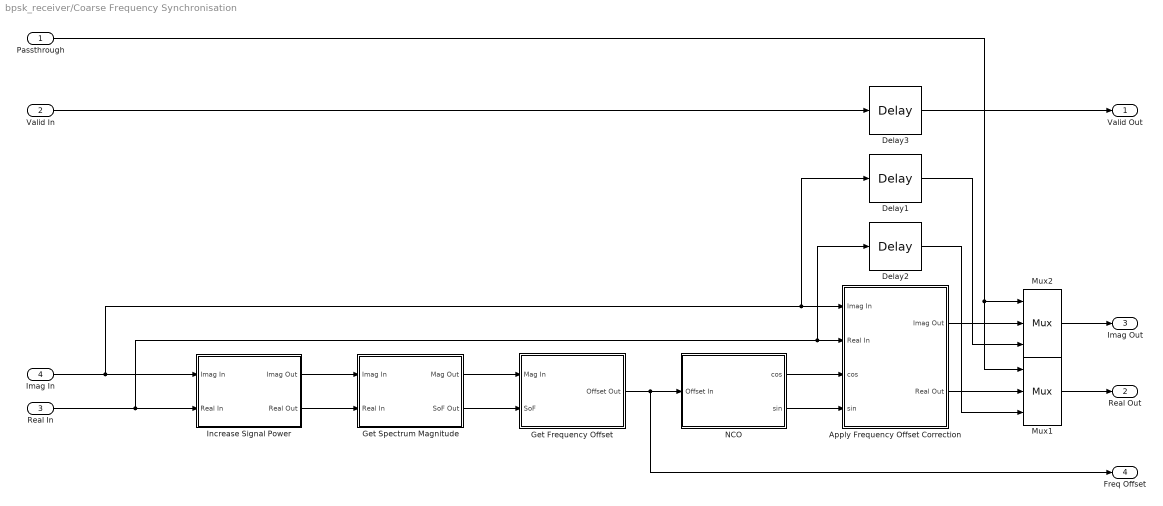
== system bpsk_receiver/Coarse Frequency Synchronisation ==
  Passthrough : Inport
  Valid In : Inport  Port=2
  Real In : Inport  Port=3
  Imag In : Inport  Port=4
  Apply Frequency Offset Correction : Subsystem
  Delay1 : xbsIndex_r4/Delay  rst=off  infoeditControl=Selection of Reset will increase slice count due to use of real FFs and instead of SRLs  en=off  latency=4  reg_retiming=off  dbl_ovrd=off  block_type=delay
  Delay2 : xbsIndex_r4/Delay  rst=off  infoeditControl=Selection of Reset will increase slice count due to use of real FFs and instead of SRLs  en=off  latency=4  reg_retiming=off  dbl_ovrd=off  block_type=delay
  Delay3 : xbsIndex_r4/Delay  rst=off  infoeditControl=Selection of Reset will increase slice count due to use of real FFs and instead of SRLs  en=off  latency=4  reg_retiming=off  dbl_ovrd=off  block_type=delay
  Get Frequency Offset : Subsystem
  Get Spectrum Magnitude : Subsystem
  Increase Signal Power : Subsystem
  Mux1 : xbsIndex_r4/Mux  inputs=2  en=off  latency=0  precision=Full  arith_type=Unsigned  n_bits=16  bin_pt=14  quantization=Truncate  overflow=Wrap  dbl_ovrd=off  block_type=mux
  Mux2 : xbsIndex_r4/Mux  inputs=2  en=off  latency=0  precision=Full  arith_type=Unsigned  n_bits=16  bin_pt=14  quantization=Truncate  overflow=Wrap  dbl_ovrd=off  block_type=mux
  NCO : Subsystem  mask(Numerically Controller Oscillator (NCO)){fs=12.8e6, n=11, L=16}
      mask prompts: fs "Sampling frequency"; n "Lookup table address size"; L "Precision of output (total bits, 2 of which integer)"
      mask help: Parameteristable NCO producing sine and cosine outputs.
      mask init:
      | N = 2^n;    % size (depth) of lookup table
      | 
      | i = ceil(log2(ceil(N/fs)))+1;   % calculate integer and fractional bits
      | b = 32-i;                         % required for constant (in conversion to step size)
  Valid Out : Outport  VectorParamsAs1DForOutWhenUnconnected=off
  Real Out : Outport  Port=2  VectorParamsAs1DForOutWhenUnconnected=off
  Imag Out : Outport  Port=3  VectorParamsAs1DForOutWhenUnconnected=off
  Freq Offset : Outport  Port=4  VectorParamsAs1DForOutWhenUnconnected=off
  wires:
  Increase Signal Power/2(Real Out) -> Get Spectrum Magnitude/2(Real In)
  NCO/1(cos) -> Apply Frequency Offset Correction/3(cos)
  Get Frequency Offset/1(Offset Out) -> Freq Offset/1, NCO/1(Offset In)
  NCO/2(sin) -> Apply Frequency Offset Correction/4(sin)
  Get Spectrum Magnitude/1(Mag Out) -> Get Frequency Offset/1(Mag In)
  Increase Signal Power/1(Imag Out) -> Get Spectrum Magnitude/1(Imag In)
  Get Spectrum Magnitude/2(SoF Out) -> Get Frequency Offset/2(SoF)
  Imag In/1 -> Increase Signal Power/1(Imag In), Delay1/1, Apply Frequency Offset Correction/1(Imag In)
  Real In/1 -> Delay2/1, Apply Frequency Offset Correction/2(Real In), Increase Signal Power/2(Real In)
  Valid In/1 -> Delay3/1
  Delay3/1 -> Valid Out/1
  Apply Frequency Offset Correction/1(Imag Out) -> Mux2/2
  Mux2/1 -> Imag Out/1
  Passthrough/1 -> Mux1/1, Mux2/1
  Mux1/1 -> Real Out/1
  Apply Frequency Offset Correction/2(Real Out) -> Mux1/2
  Delay1/1 -> Mux2/3
  Delay2/1 -> Mux1/3

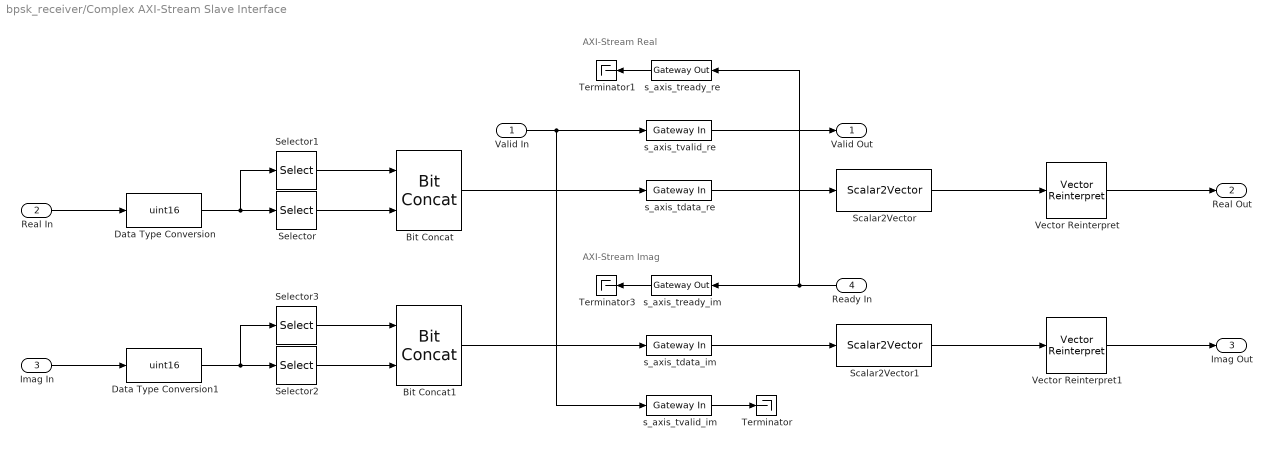
== system bpsk_receiver/Complex AXI-Stream Slave Interface ==
  note: AXI-Stream Real
  note: AXI-Stream Imag
  Valid In : Inport
  Real In : Inport  Port=2
  Imag In : Inport  Port=3
  Ready In : Inport  Port=4
  Bit Concat : hdlsllib/Logic and Bit Operations/Bit Concat  numInputs=2
  Bit Concat1 : hdlsllib/Logic and Bit Operations/Bit Concat  numInputs=2
  Data Type Conversion : DataTypeConversion  OutDataTypeStr=uint16  ConvertRealWorld=Stored Integer (SI)
  Data Type Conversion1 : DataTypeConversion  OutDataTypeStr=uint16  ConvertRealWorld=Stored Integer (SI)
  Scalar2Vector : xrbsSSR_Library/Scalar2Vector  Width=16  sg_ssr=2  sg_ssr_prev=2  sg_ssr_name=vect_Scalar2Vector  block_type=scalar2vector_ssr
      settings: SourceProductName=Xilinx SSR Blockset
  Scalar2Vector1 : xrbsSSR_Library/Scalar2Vector  Width=16  sg_ssr=2  sg_ssr_prev=2  sg_ssr_name=vect_Scalar2Vector  block_type=scalar2vector_ssr
      settings: SourceProductName=Xilinx SSR Blockset
  Selector : Selector  NumberOfDimensions=2  IndexMode=Zero-based  InputPortWidth=3  IndexOptions=Index vector (dialog),Index vector (dialog)  Indices=0,0  OutputSizes=1,1
  Selector1 : Selector  NumberOfDimensions=2  IndexMode=Zero-based  InputPortWidth=3  IndexOptions=Index vector (dialog),Index vector (dialog)  Indices=1,0  OutputSizes=1,1
  Selector2 : Selector  NumberOfDimensions=2  IndexMode=Zero-based  InputPortWidth=3  IndexOptions=Index vector (dialog),Index vector (dialog)  Indices=0,0  OutputSizes=1,1
  Selector3 : Selector  NumberOfDimensions=2  IndexMode=Zero-based  InputPortWidth=3  IndexOptions=Index vector (dialog),Index vector (dialog)  Indices=1,0  OutputSizes=1,1
  Terminator : Terminator
  Terminator1 : Terminator
  Terminator3 : Terminator
  Vector Reinterpret : xrbsSSR_Library/Vector Reinterpret  sg_ssr=2  sg_ssr_prev=2  force_arith_type=on  arith_type="Signed  (2's comp)"  force_bin_pt=on  bin_pt=14  block_type=reinterpret_ssr
      settings: SourceProductName=Xilinx SSR Blockset  infoedit="The Vector Reinterpret block Changes vector input signal type without altering the binary representation. You can change the signal between signed and unsigned, and relocate the binary point.<br><br>Hardware notes: In hardware this block costs nothing.<br><br>Example:  Suppose the input is 6 bits wide, signed, with 2 fractional bits, and the output is forced to unsigned with 0 fractional bits.  Then an input of -2.0 (1110.00 in binary 2's complement) becomes an output of 56 (111000 in binary)."
  Vector Reinterpret1 : xrbsSSR_Library/Vector Reinterpret  sg_ssr=2  sg_ssr_prev=2  force_arith_type=on  arith_type="Signed  (2's comp)"  force_bin_pt=on  bin_pt=14  block_type=reinterpret_ssr
      settings: SourceProductName=Xilinx SSR Blockset  infoedit="The Vector Reinterpret block Changes vector input signal type without altering the binary representation. You can change the signal between signed and unsigned, and relocate the binary point.<br><br>Hardware notes: In hardware this block costs nothing.<br><br>Example:  Suppose the input is 6 bits wide, signed, with 2 fractional bits, and the output is forced to unsigned with 0 fractional bits.  Then an input of -2.0 (1110.00 in binary 2's complement) becomes an output of 56 (111000 in binary)."
  s_axis_tdata_im : xbsIndex_r4/Gateway In  gui_display_data_type=Fixed-point  arith_type=Unsigned  n_bits=32  bin_pt=0  preci_type=Single  exp_width=8  frac_width=24  rows=1  columns=1  quantization="Round  (unbiased: +/- Inf)"  overflow=Saturate  period=1/64e6  UseAsADC=off  ADCChannel='1'  interface=None  automatic_assignment=on  address_offset=hex2dec('00')  intf_name=''  intf_description=''  default_value=0  timing_constraint=None  locs_specified=off  LOCs={}  io_standard={}  inherit_from_input=off  hdl_port=on  dbl_ovrd=off  block_type=gatewayin
  s_axis_tdata_re : xbsIndex_r4/Gateway In  gui_display_data_type=Fixed-point  arith_type=Unsigned  n_bits=32  bin_pt=0  preci_type=Single  exp_width=8  frac_width=24  rows=1  columns=1  quantization="Round  (unbiased: +/- Inf)"  overflow=Saturate  period=1/64e6  UseAsADC=off  ADCChannel='1'  interface=None  automatic_assignment=on  address_offset=hex2dec('00')  intf_name=''  intf_description=''  default_value=0  timing_constraint=None  locs_specified=off  LOCs={}  io_standard={}  inherit_from_input=off  hdl_port=on  dbl_ovrd=off  block_type=gatewayin
  s_axis_tready_im : xbsIndex_r4/Gateway Out  inherit_from_input=off  hdl_port=on  rows=1  columns=1  UseAsDAC=off  DACChannel='1'  interface=None  automatic_assignment=on  address_offset=hex2dec('00')  intf_name=''  intf_description=''  timing_constraint=None  locs_specified=off  LOCs={}  io_standard={}  block_type=gatewayout
  s_axis_tready_re : xbsIndex_r4/Gateway Out  inherit_from_input=off  hdl_port=on  rows=1  columns=1  UseAsDAC=off  DACChannel='1'  interface=None  automatic_assignment=on  address_offset=hex2dec('00')  intf_name=''  intf_description=''  timing_constraint=None  locs_specified=off  LOCs={}  io_standard={}  block_type=gatewayout
  s_axis_tvalid_im : xbsIndex_r4/Gateway In  gui_display_data_type=Boolean  arith_type=Boolean  n_bits=16  bin_pt=14  preci_type=Single  exp_width=8  frac_width=24  rows=1  columns=1  quantization="Round  (unbiased: +/- Inf)"  overflow=Saturate  period=1/64e6  UseAsADC=off  ADCChannel='1'  interface=None  automatic_assignment=on  address_offset=hex2dec('00')  intf_name=''  intf_description=''  default_value=0  timing_constraint=None  locs_specified=off  LOCs={}  io_standard={}  inherit_from_input=off  hdl_port=on  dbl_ovrd=off  block_type=gatewayin
  s_axis_tvalid_re : xbsIndex_r4/Gateway In  gui_display_data_type=Boolean  arith_type=Boolean  n_bits=16  bin_pt=14  preci_type=Single  exp_width=8  frac_width=24  rows=1  columns=1  quantization="Round  (unbiased: +/- Inf)"  overflow=Saturate  period=1/64e6  UseAsADC=off  ADCChannel='1'  interface=None  automatic_assignment=on  address_offset=hex2dec('00')  intf_name=''  intf_description=''  default_value=0  timing_constraint=None  locs_specified=off  LOCs={}  io_standard={}  inherit_from_input=off  hdl_port=on  dbl_ovrd=off  block_type=gatewayin
  Valid Out : Outport  VectorParamsAs1DForOutWhenUnconnected=off
  Real Out : Outport  Port=2  VectorParamsAs1DForOutWhenUnconnected=off
  Imag Out : Outport  Port=3  VectorParamsAs1DForOutWhenUnconnected=off
  wires:
  s_axis_tready_re/1 -> Terminator1/1
  s_axis_tdata_re/1 -> Scalar2Vector/1
  Valid In/1 -> s_axis_tvalid_re/1, s_axis_tvalid_im/1
  Ready In/1 -> s_axis_tready_im/1, s_axis_tready_re/1
  s_axis_tvalid_re/1 -> Valid Out/1
  s_axis_tvalid_im/1 -> Terminator/1
  s_axis_tready_im/1 -> Terminator3/1
  Scalar2Vector/1 -> Vector Reinterpret/1
  Real In/1 -> Data Type Conversion/1
  Data Type Conversion/1 -> Selector1/1, Selector/1
  Bit Concat/1 -> s_axis_tdata_re/1
  Selector/1 -> Bit Concat/2
  Selector1/1 -> Bit Concat/1
  Vector Reinterpret/1 -> Real Out/1
  Selector3/1 -> Bit Concat1/1
  Selector2/1 -> Bit Concat1/2
  Bit Concat1/1 -> s_axis_tdata_im/1
  Data Type Conversion1/1 -> Selector2/1, Selector3/1
  Imag In/1 -> Data Type Conversion1/1
  Vector Reinterpret1/1 -> Imag Out/1
  Scalar2Vector1/1 -> Vector Reinterpret1/1
  s_axis_tdata_im/1 -> Scalar2Vector1/1
